simulink model "untitled4"  (R2024b)
settings: Solver=VariableStepAuto  StartTime=0.0  StopTime=300  RelTol=1e-3
values from neighbouring files (symbols this model uses):
  R = 0.246    [Ex_6.m]
undefined symbols (not defined in the file or in its folder): denC, denG, numC, numG
settings Model: Creator=EdoPolito  LastModifiedBy=EdoPolito

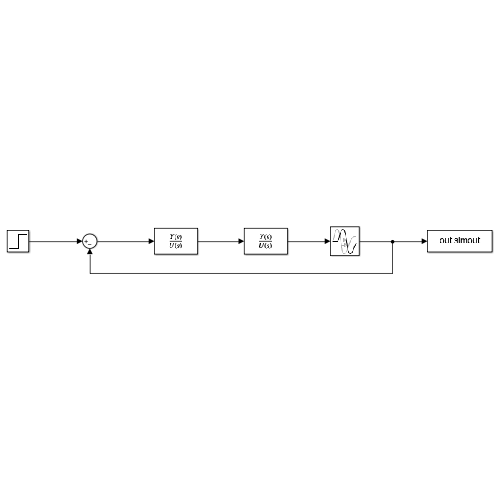
[thumbnail: Simulink's stored preview of the top-level diagram]
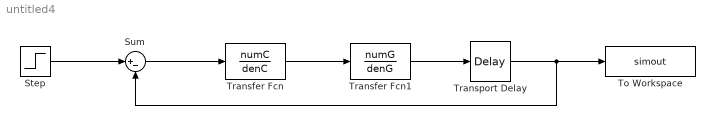
== system untitled4 ==
  Step : Step  SampleTime=0
  Sum : Sum  Inputs=|+-
  To Workspace : ToWorkspace  VariableName=simout  SaveFormat=Timeseries  SampleTime=-1
  Transfer Fcn : TransferFcn  Numerator=numC  Denominator=denC
  Transfer Fcn1 : TransferFcn  Numerator=numG  Denominator=denG
  Transport Delay : TransportDelay  DelayTime=R
  wires:
  Step/1 -> Sum/1
  Sum/1 -> Transfer Fcn/1
  Transfer Fcn/1 -> Transfer Fcn1/1
  Transfer Fcn1/1 -> Transport Delay/1
  Transport Delay/1 -> Sum/2, To Workspace/1
